simulink model "test_qdr_vacc4"  (Simulink 7.2)
settings: Solver=ode45  StartTime=0.0  StopTime=400000  RelTol=1e-3
libraries: xbsIndex_r4 x317, xps_library x15, casper_library_misc x4, casper_library_scopes x1
(part 2 of 3)

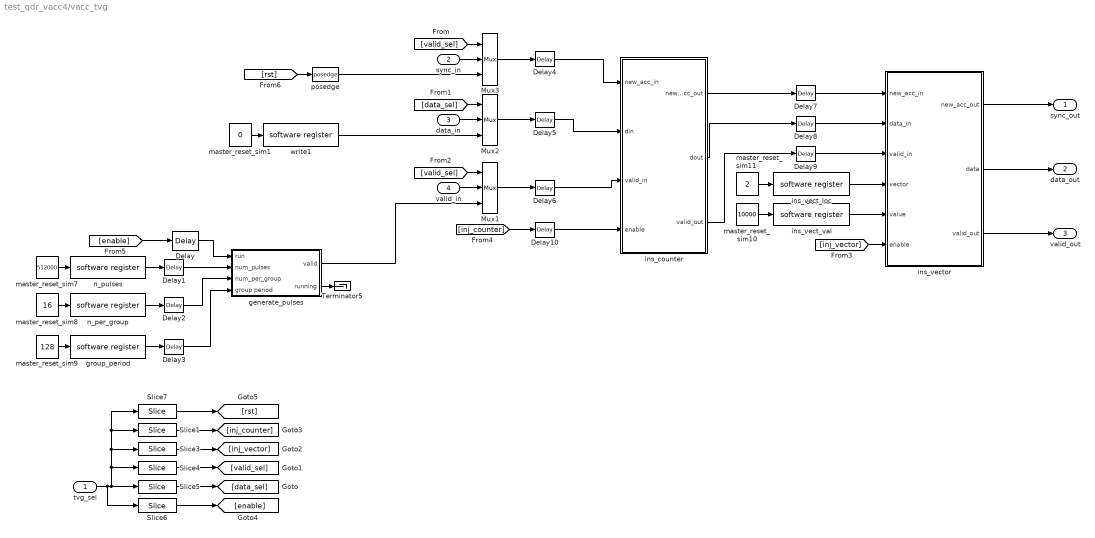
== system test_qdr_vacc4/vacc_tvg ==
  tvg_sel : Inport  OutDataType=sfix(16)  OutScaling=2^0
  sync_in : Inport  Port=2  OutDataType=sfix(16)  OutScaling=2^0
  data_in : Inport  Port=3  OutDataType=sfix(16)  OutScaling=2^0
  valid_in : Inport  Port=4  OutDataType=sfix(16)  OutScaling=2^0
  Delay : xbsIndex_r4/Delay  en=off  latency=1  dbl_ovrd=off  reg_retiming=on  block_type=delay
      settings: xl_area=[0, 0, 0, 0, 0, 0, 0]
  Delay{1..10} (10 alike) : xbsIndex_r4/Delay  en=off  latency=2  dbl_ovrd=off  reg_retiming=on  block_type=delay
  Mux1 : xbsIndex_r4/Mux  inputs=2  en=off  latency=0  precision=Full  arith_type="Signed  (2's comp)"  n_bits=8  bin_pt=2  quantization=Truncate  overflow=Wrap  dbl_ovrd=off  block_type=mux
      settings: xl_area=[0, 0, 0, 0, 0, 0, 0]
  Mux2 : xbsIndex_r4/Mux  inputs=2  en=off  latency=0  precision=Full  arith_type="Signed  (2's comp)"  n_bits=8  bin_pt=2  quantization=Truncate  overflow=Wrap  dbl_ovrd=off  block_type=mux
      settings: xl_area=[0, 0, 0, 0, 0, 0, 0]
  Mux3 : xbsIndex_r4/Mux  inputs=2  en=off  latency=0  precision=Full  arith_type="Signed  (2's comp)"  n_bits=8  bin_pt=2  quantization=Truncate  overflow=Wrap  dbl_ovrd=off  block_type=mux
      settings: xl_area=[0, 0, 0, 0, 0, 0, 0]
  Slice1 : xbsIndex_r4/Slice  nbits=1  boolean_output=on  mode=Lower Bit Location + Width  bit1=0  base1=MSB of Input  bit0=4  base0=LSB of Input  dbl_ovrd=off  block_type=slice
      settings: infoedit="Extracts a given range of bits from each input sample and presents it at the output.  The output type is ordinarily unsigned with binary point at zero, but can be Boolean when the slice is one bit wide.<P><P>Hardware notes: In hardware this block costs nothing."  block_version=10.1.3
  Slice3 : xbsIndex_r4/Slice  nbits=1  boolean_output=on  mode=Lower Bit Location + Width  bit1=0  base1=MSB of Input  bit0=3  base0=LSB of Input  dbl_ovrd=off  block_type=slice
      settings: infoedit="Extracts a given range of bits from each input sample and presents it at the output.  The output type is ordinarily unsigned with binary point at zero, but can be Boolean when the slice is one bit wide.<P><P>Hardware notes: In hardware this block costs nothing."  block_version=10.1.3
  Slice4 : xbsIndex_r4/Slice  nbits=1  boolean_output=on  mode=Lower Bit Location + Width  bit1=0  base1=MSB of Input  bit0=2  base0=LSB of Input  dbl_ovrd=off  block_type=slice
      settings: infoedit="Extracts a given range of bits from each input sample and presents it at the output.  The output type is ordinarily unsigned with binary point at zero, but can be Boolean when the slice is one bit wide.<P><P>Hardware notes: In hardware this block costs nothing."  block_version=10.1.3
  Slice5 : xbsIndex_r4/Slice  nbits=1  boolean_output=on  mode=Lower Bit Location + Width  bit1=0  base1=MSB of Input  bit0=1  base0=LSB of Input  dbl_ovrd=off  block_type=slice
      settings: infoedit="Extracts a given range of bits from each input sample and presents it at the output.  The output type is ordinarily unsigned with binary point at zero, but can be Boolean when the slice is one bit wide.<P><P>Hardware notes: In hardware this block costs nothing."  block_version=10.1.3
  Slice6 : xbsIndex_r4/Slice  nbits=1  boolean_output=on  mode=Lower Bit Location + Width  bit1=0  base1=MSB of Input  bit0=0  base0=LSB of Input  dbl_ovrd=off  block_type=slice
      settings: infoedit="Extracts a given range of bits from each input sample and presents it at the output.  The output type is ordinarily unsigned with binary point at zero, but can be Boolean when the slice is one bit wide.<P><P>Hardware notes: In hardware this block costs nothing."  block_version=10.1.3
  Slice7 : xbsIndex_r4/Slice  nbits=1  boolean_output=on  mode=Lower Bit Location + Width  bit1=0  base1=MSB of Input  bit0=5  base0=LSB of Input  dbl_ovrd=off  block_type=slice
      settings: infoedit="Extracts a given range of bits from each input sample and presents it at the output.  The output type is ordinarily unsigned with binary point at zero, but can be Boolean when the slice is one bit wide.<P><P>Hardware notes: In hardware this block costs nothing."  block_version=10.1.3
  Terminator5 : Terminator
  generate_pulses : Subsystem
  group_period : xps_library/software register  Tag=xps:sw_reg  SystemSampleTime=-1  io_dir=From Processor  arith_type=Unsigned  bitwidth=32  bin_pt=0  sample_period=1  gw_name=test_qdr_vacc4_vacc_tvg_group_period_user_data_out
      link override qdr_vacc_dram_tvg1_group_period_user_data_out: arith_type=Unsigned  n_bits=32  bin_pt=0  period=1
      link override qdr_vacc_qdr_tvg_group_period_user_data_out: arith_type=Unsigned  n_bits=32  bin_pt=0  period=1
      link override test_d_v_p_10_1_new_packet_format_qdr_tvg_group_period_user_data_out: arith_type=Unsigned  n_bits=32  bin_pt=0  period=1
      link override test_qdr_vacc2_vacc_tvg_group_period_user_data_out: arith_type=Unsigned  n_bits=32  bin_pt=0  period=1
      link override test_qdr_vacc3_vacc_tvg_group_period_user_data_out: arith_type=Unsigned  n_bits=32  bin_pt=0  period=1
      link override test_qdr_vacc_qdr_tvg_group_period_user_data_out: arith_type=Unsigned  n_bits=32  bin_pt=0  period=1
      link override test_qdr_vacc_vacc_tvg_group_period_user_data_out: arith_type=Unsigned  n_bits=32  bin_pt=0  period=1
      link override test_vacc_10_1_new_pkt_form_qdr_tvg_group_period_user_data_out: arith_type=Unsigned  n_bits=32  bin_pt=0  period=1
      link override test_vacc_pkt_10_1_vacc_tvg0_group_period_user_data_out: arith_type=Unsigned  n_bits=32  bin_pt=0  period=1
      link override test_vacc_pkt_10_1_vacc_tvg_group_period_user_data_out: arith_type=Unsigned  n_bits=32  bin_pt=0  period=1
      link override xflow_sim_8a_vacc_tvg0_group_period_user_data_out: arith_type=Unsigned  n_bits=32  bin_pt=0  period=1
      link override xflow_sim_vacc_tvg0_group_period_user_data_out: arith_type=Unsigned  n_bits=32  bin_pt=0  period=1
  ins_counter : Subsystem  mask{vec_len=len}
      mask prompts: vec_len "Vector Length?"
      mask init:
      | fmtstr = sprintf('Vector Length: %d', vec_len);
      | set_param(gcb, 'AttributesFormatString', fmtstr);
      settings: AttributesFormatString=Vector Length: 1000
  ins_vect_loc : xps_library/software register  Tag=xps:sw_reg  SystemSampleTime=-1  io_dir=From Processor  arith_type=Unsigned  bitwidth=32  bin_pt=0  sample_period=1  gw_name=test_qdr_vacc4_vacc_tvg_ins_vect_loc_user_data_out
      link override qdr_vacc_dram_tvg1_inject_vector_location_user_data_out: arith_type=Unsigned  n_bits=32  bin_pt=0  period=1
      link override qdr_vacc_qdr_tvg_inject_vector_location_user_data_out: arith_type=Unsigned  n_bits=32  bin_pt=0  period=1
      link override test_d_v_p_10_1_new_packet_format_qdr_tvg_inject_vector_location_user_data_out: arith_type=Unsigned  n_bits=32  bin_pt=0  period=1
      link override test_qdr_vacc2_vacc_tvg_ins_vect_loc_user_data_out: arith_type=Unsigned  n_bits=32  bin_pt=0  period=1
      link override test_qdr_vacc3_vacc_tvg_ins_vect_loc_user_data_out: arith_type=Unsigned  n_bits=32  bin_pt=0  period=1
      link override test_qdr_vacc_qdr_tvg_inject_vector_location_user_data_out: arith_type=Unsigned  n_bits=32  bin_pt=0  period=1
      link override test_qdr_vacc_vacc_tvg_ins_vect_loc_user_data_out: arith_type=Unsigned  n_bits=32  bin_pt=0  period=1
      link override test_vacc_10_1_new_pkt_form_qdr_tvg_inject_vector_location_user_data_out: arith_type=Unsigned  n_bits=32  bin_pt=0  period=1
      link override test_vacc_pkt_10_1_vacc_tvg0_ins_vect_loc_user_data_out: arith_type=Unsigned  n_bits=32  bin_pt=0  period=1
      link override test_vacc_pkt_10_1_vacc_tvg_inject_vector_location_user_data_out: arith_type=Unsigned  n_bits=32  bin_pt=0  period=1
      link override test_vacc_pkt_10_1_vacc_tvg_ins_vect_loc_user_data_out: arith_type=Unsigned  n_bits=32  bin_pt=0  period=1
      link override xflow_sim_8a_vacc_tvg0_ins_vect_loc_user_data_out: arith_type=Unsigned  n_bits=32  bin_pt=0  period=1
      link override xflow_sim_vacc_tvg0_ins_vect_loc_user_data_out: arith_type=Unsigned  n_bits=32  bin_pt=0  period=1
  ins_vect_val : xps_library/software register  Tag=xps:sw_reg  SystemSampleTime=-1  io_dir=From Processor  arith_type=Unsigned  bitwidth=32  bin_pt=0  sample_period=1  gw_name=test_qdr_vacc4_vacc_tvg_ins_vect_val_user_data_out
      link override qdr_vacc_dram_tvg1_inject_vector_value_user_data_out: arith_type=Unsigned  n_bits=32  bin_pt=0  period=1
      link override qdr_vacc_qdr_tvg_inject_vector_value_user_data_out: arith_type=Unsigned  n_bits=32  bin_pt=0  period=1
      link override test_d_v_p_10_1_new_packet_format_qdr_tvg_inject_vector_value_user_data_out: arith_type="Signed  (2's comp)"  n_bits=32  bin_pt=0  period=1
      link override test_qdr_vacc2_vacc_tvg_ins_vect_val_user_data_out: arith_type=Unsigned  n_bits=32  bin_pt=0  period=1
      link override test_qdr_vacc3_vacc_tvg_ins_vect_val_user_data_out: arith_type=Unsigned  n_bits=32  bin_pt=0  period=1
      link override test_qdr_vacc_qdr_tvg_inject_vector_value_user_data_out: arith_type="Signed  (2's comp)"  n_bits=32  bin_pt=0  period=1
      link override test_qdr_vacc_vacc_tvg_ins_vect_val_user_data_out: arith_type=Unsigned  n_bits=32  bin_pt=0  period=1
      link override test_vacc_10_1_new_pkt_form_qdr_tvg_inject_vector_value_user_data_out: arith_type="Signed  (2's comp)"  n_bits=32  bin_pt=0  period=1
      link override test_vacc_pkt_10_1_vacc_tvg0_ins_vect_val_user_data_out: arith_type=Unsigned  n_bits=32  bin_pt=0  period=1
      link override test_vacc_pkt_10_1_vacc_tvg_inject_vector_value_user_data_out: arith_type="Signed  (2's comp)"  n_bits=32  bin_pt=0  period=1
      link override test_vacc_pkt_10_1_vacc_tvg_ins_vect_val_user_data_out: arith_type="Signed  (2's comp)"  n_bits=32  bin_pt=0  period=1
      link override xflow_sim_8a_vacc_tvg0_ins_vect_val_user_data_out: arith_type=Unsigned  n_bits=32  bin_pt=0  period=1
      link override xflow_sim_vacc_tvg0_ins_vect_val_user_data_out: arith_type=Unsigned  n_bits=32  bin_pt=0  period=1
  ins_vector : Subsystem  mask{num_vectors=len}
      mask prompts: num_vectors "number of vectors"
      mask init:
      | fmtstr = sprintf('Vector Length: %d', num_vectors);
      | set_param(gcb, 'AttributesFormatString', fmtstr);
      settings: AttributesFormatString=Vector Length: 1000
  master_reset_sim1 : Constant  Value=0  OutDataType=sfix(16)  OutScaling=2^0
  master_reset_sim10 : Constant  Value=10000  OutDataType=sfix(16)  OutScaling=2^0
  master_reset_sim11 : Constant  Value=2  OutDataType=sfix(16)  OutScaling=2^0
  master_reset_sim7 : Constant  Value=512000  OutDataType=sfix(16)  OutScaling=2^0
  master_reset_sim8 : Constant  Value=16  OutDataType=sfix(16)  OutScaling=2^0
  master_reset_sim9 : Constant  Value=128  OutDataType=sfix(16)  OutScaling=2^0
  n_per_group : xps_library/software register  Tag=xps:sw_reg  SystemSampleTime=-1  io_dir=From Processor  arith_type=Unsigned  bitwidth=32  bin_pt=0  sample_period=1  gw_name=test_qdr_vacc4_vacc_tvg_n_per_group_user_data_out
      link override qdr_vacc_dram_tvg1_num_per_group_user_data_out: arith_type=Unsigned  n_bits=32  bin_pt=0  period=1
      link override qdr_vacc_qdr_tvg_num_per_group_user_data_out: arith_type=Unsigned  n_bits=32  bin_pt=0  period=1
      link override test_d_v_p_10_1_new_packet_format_qdr_tvg_num_per_group_user_data_out: arith_type=Unsigned  n_bits=32  bin_pt=0  period=1
      link override test_qdr_vacc2_vacc_tvg_n_per_group_user_data_out: arith_type=Unsigned  n_bits=32  bin_pt=0  period=1
      link override test_qdr_vacc3_vacc_tvg_n_per_group_user_data_out: arith_type=Unsigned  n_bits=32  bin_pt=0  period=1
      link override test_qdr_vacc_qdr_tvg_num_per_group_user_data_out: arith_type=Unsigned  n_bits=32  bin_pt=0  period=1
      link override test_qdr_vacc_vacc_tvg_n_per_group_user_data_out: arith_type=Unsigned  n_bits=32  bin_pt=0  period=1
      link override test_vacc_10_1_new_pkt_form_qdr_tvg_num_per_group_user_data_out: arith_type=Unsigned  n_bits=32  bin_pt=0  period=1
      link override test_vacc_pkt_10_1_vacc_tvg0_num_per_group_user_data_out: arith_type=Unsigned  n_bits=32  bin_pt=0  period=1
      link override test_vacc_pkt_10_1_vacc_tvg_num_per_group_user_data_out: arith_type=Unsigned  n_bits=32  bin_pt=0  period=1
      link override xflow_sim_8a_vacc_tvg0_num_per_group_user_data_out: arith_type=Unsigned  n_bits=32  bin_pt=0  period=1
      link override xflow_sim_vacc_tvg0_num_per_group_user_data_out: arith_type=Unsigned  n_bits=32  bin_pt=0  period=1
  n_pulses : xps_library/software register  Tag=xps:sw_reg  SystemSampleTime=-1  io_dir=From Processor  arith_type=Unsigned  bitwidth=32  bin_pt=0  sample_period=1  gw_name=test_qdr_vacc4_vacc_tvg_n_pulses_user_data_out
      link override qdr_vacc_dram_tvg1_num_pulses_user_data_out: arith_type=Unsigned  n_bits=32  bin_pt=0  period=1
      link override qdr_vacc_qdr_tvg_num_pulses_user_data_out: arith_type=Unsigned  n_bits=32  bin_pt=0  period=1
      link override test_d_v_p_10_1_new_packet_format_qdr_tvg_num_pulses_user_data_out: arith_type=Unsigned  n_bits=32  bin_pt=0  period=1
      link override test_qdr_vacc2_vacc_tvg_n_pulses_user_data_out: arith_type=Unsigned  n_bits=32  bin_pt=0  period=1
      link override test_qdr_vacc3_vacc_tvg_n_pulses_user_data_out: arith_type=Unsigned  n_bits=32  bin_pt=0  period=1
      link override test_qdr_vacc_qdr_tvg_num_pulses_user_data_out: arith_type=Unsigned  n_bits=32  bin_pt=0  period=1
      link override test_qdr_vacc_vacc_tvg_n_pulses_user_data_out: arith_type=Unsigned  n_bits=32  bin_pt=0  period=1
      link override test_vacc_10_1_new_pkt_form_qdr_tvg_num_pulses_user_data_out: arith_type=Unsigned  n_bits=32  bin_pt=0  period=1
      link override test_vacc_pkt_10_1_vacc_tvg0_num_pulses_user_data_out: arith_type=Unsigned  n_bits=32  bin_pt=0  period=1
      link override test_vacc_pkt_10_1_vacc_tvg_num_pulses_user_data_out: arith_type=Unsigned  n_bits=32  bin_pt=0  period=1
      link override xflow_sim_8a_vacc_tvg0_num_pulses_user_data_out: arith_type=Unsigned  n_bits=32  bin_pt=0  period=1
      link override xflow_sim_vacc_tvg0_num_pulses_user_data_out: arith_type=Unsigned  n_bits=32  bin_pt=0  period=1
  posedge : casper_library_misc/posedge  Tag=Rising Edge Detector  SystemSampleTime=-1
  write1 : xps_library/software register  Tag=xps:sw_reg  SystemSampleTime=-1  io_dir=From Processor  arith_type=Unsigned  bitwidth=32  bin_pt=0  sample_period=1  gw_name=test_qdr_vacc4_vacc_tvg_write1_user_data_out
      link override qdr_vacc_dram_tvg1_write1_user_data_out: arith_type=Unsigned  n_bits=32  bin_pt=0  period=1
      link override qdr_vacc_qdr_tvg_write1_user_data_out: arith_type=Unsigned  n_bits=32  bin_pt=0  period=1
      link override test_d_v_p_10_1_new_packet_format_qdr_tvg_write1_user_data_out: arith_type="Signed  (2's comp)"  n_bits=32  bin_pt=0  period=1
      link override test_qdr_vacc2_vacc_tvg_write1_user_data_out: arith_type=Unsigned  n_bits=32  bin_pt=0  period=1
      link override test_qdr_vacc3_vacc_tvg_write1_user_data_out: arith_type=Unsigned  n_bits=32  bin_pt=0  period=1
      link override test_qdr_vacc_qdr_tvg_write1_user_data_out: arith_type="Signed  (2's comp)"  n_bits=32  bin_pt=0  period=1
      link override test_qdr_vacc_vacc_tvg_write1_user_data_out: arith_type=Unsigned  n_bits=32  bin_pt=0  period=1
      link override test_vacc_10_1_new_pkt_form_qdr_tvg_write1_user_data_out: arith_type="Signed  (2's comp)"  n_bits=32  bin_pt=0  period=1
      link override test_vacc_pkt_10_1_vacc_tvg0_write1_user_data_out: arith_type=Unsigned  n_bits=32  bin_pt=0  period=1
      link override test_vacc_pkt_10_1_vacc_tvg_write1_user_data_out: arith_type="Signed  (2's comp)"  n_bits=32  bin_pt=0  period=1
      link override xflow_sim_8a_vacc_tvg0_write1_user_data_out: arith_type=Unsigned  n_bits=32  bin_pt=0  period=1
      link override xflow_sim_vacc_tvg0_write1_user_data_out: arith_type=Unsigned  n_bits=32  bin_pt=0  period=1
  sync_out : Outport  OutDataType=sfix(16)  OutScaling=2^0
  data_out : Outport  Port=2  OutDataType=sfix(16)  OutScaling=2^0
  valid_out : Outport  Port=3  OutDataType=sfix(16)  OutScaling=2^0
  wires:
  generate_pulses/2(running) -> Terminator5/1
  Delay/1 -> generate_pulses/1(run)
  Slice7/1 -> [rst]
  Slice6/1 -> [enable]
  [inj_counter] -> Delay10/1
  ins_vect_val/1 -> ins_vector/5(value)
  master_reset_sim10/1 -> ins_vect_val/1
  ins_vect_loc/1 -> ins_vector/4(vector)
  master_reset_sim11/1 -> ins_vect_loc/1
  [inj_vector] -> ins_vector/6(enable)
  posedge/1 -> Mux3/3
  generate_pulses/1(valid) -> Mux1/3
  ins_counter/3(valid_out) -> Delay9/1
  ins_counter/2(dout) -> Delay8/1
  [enable] -> Delay/1
  Slice1/1 -> [inj_counter]
  Slice3/1 -> [inj_vector]
  [valid_sel] -> Mux1/1
  [data_sel] -> Mux2/1
  [valid_sel] -> Mux3/1
  Slice4/1 -> [valid_sel]
  tvg_sel/1 -> Slice6/1, Slice4/1, Slice7/1, Slice1/1, Slice3/1, Slice5/1
  Slice5/1 -> [data_sel]
  Mux3/1 -> Delay4/1
  sync_in/1 -> Mux3/2
  data_in/1 -> Mux2/2
  Mux2/1 -> Delay5/1
  ins_counter/1(new_acc_out) -> Delay7/1
  ins_vector/3(valid_out) -> valid_out/1
  ins_vector/2(data) -> data_out/1
  ins_vector/1(new_acc_out) -> sync_out/1
  valid_in/1 -> Mux1/2
  Mux1/1 -> Delay6/1
  master_reset_sim9/1 -> group_period/1
  group_period/1 -> Delay3/1
  master_reset_sim8/1 -> n_per_group/1
  n_per_group/1 -> Delay2/1
  master_reset_sim7/1 -> n_pulses/1
  n_pulses/1 -> Delay1/1
  [rst] -> posedge/1
  master_reset_sim1/1 -> write1/1
  write1/1 -> Mux2/3
  Delay1/1 -> generate_pulses/2(num_pulses)
  Delay2/1 -> generate_pulses/3(num_per_group)
  Delay3/1 -> generate_pulses/4(group period)
  Delay4/1 -> ins_counter/1(new_acc_in)
  Delay5/1 -> ins_counter/2(din)
  Delay6/1 -> ins_counter/3(valid_in)
  Delay7/1 -> ins_vector/1(new_acc_in)
  Delay8/1 -> ins_vector/2(data_in)
  Delay9/1 -> ins_vector/3(valid_in)
  Delay10/1 -> ins_counter/4(enable)

== system test_qdr_vacc4/Subsystem/data_sel1 ==
  In1 : Inport  OutDataType=sfix(16)  OutScaling=2^0
  Product : Product  OutDataType=sfix(16)  OutScaling=2^0  RndMeth=Zero
  err_clear_sim1 : Constant  Value=2^bit_pos  OutDataType=sfix(16)  OutScaling=2^0
  Out1 : Outport  OutDataType=sfix(16)  OutScaling=2^0
  wires:
  err_clear_sim1/1 -> Product/2
  In1/1 -> Product/1
  Product/1 -> Out1/1

== system test_qdr_vacc4/Subsystem/inj_counter1 ==
  In1 : Inport  OutDataType=sfix(16)  OutScaling=2^0
  Product : Product  OutDataType=sfix(16)  OutScaling=2^0  RndMeth=Zero
  err_clear_sim1 : Constant  Value=2^bit_pos  OutDataType=sfix(16)  OutScaling=2^0
  Out1 : Outport  OutDataType=sfix(16)  OutScaling=2^0
  wires:
  err_clear_sim1/1 -> Product/2
  In1/1 -> Product/1
  Product/1 -> Out1/1

== system test_qdr_vacc4/Subsystem/inj_vector1 ==
  In1 : Inport  OutDataType=sfix(16)  OutScaling=2^0
  Product : Product  OutDataType=sfix(16)  OutScaling=2^0  RndMeth=Zero
  err_clear_sim1 : Constant  Value=2^bit_pos  OutDataType=sfix(16)  OutScaling=2^0
  Out1 : Outport  OutDataType=sfix(16)  OutScaling=2^0
  wires:
  err_clear_sim1/1 -> Product/2
  In1/1 -> Product/1
  Product/1 -> Out1/1

== system test_qdr_vacc4/Subsystem/new_acc2 ==
  In1 : Inport  OutDataType=sfix(16)  OutScaling=2^0
  Product : Product  OutDataType=sfix(16)  OutScaling=2^0  RndMeth=Zero
  err_clear_sim1 : Constant  Value=2^bit_pos  OutDataType=sfix(16)  OutScaling=2^0
  Out1 : Outport  OutDataType=sfix(16)  OutScaling=2^0
  wires:
  err_clear_sim1/1 -> Product/2
  In1/1 -> Product/1
  Product/1 -> Out1/1

== system test_qdr_vacc4/Subsystem/run1 ==
  In1 : Inport  OutDataType=sfix(16)  OutScaling=2^0
  Product : Product  OutDataType=sfix(16)  OutScaling=2^0  RndMeth=Zero
  err_clear_sim1 : Constant  Value=2^bit_pos  OutDataType=sfix(16)  OutScaling=2^0
  Out1 : Outport  OutDataType=sfix(16)  OutScaling=2^0
  wires:
  err_clear_sim1/1 -> Product/2
  In1/1 -> Product/1
  Product/1 -> Out1/1

== system test_qdr_vacc4/Subsystem/valid_sel1 ==
  In1 : Inport  OutDataType=sfix(16)  OutScaling=2^0
  Product : Product  OutDataType=sfix(16)  OutScaling=2^0  RndMeth=Zero
  err_clear_sim1 : Constant  Value=2^bit_pos  OutDataType=sfix(16)  OutScaling=2^0
  Out1 : Outport  OutDataType=sfix(16)  OutScaling=2^0
  wires:
  err_clear_sim1/1 -> Product/2
  In1/1 -> Product/1
  Product/1 -> Out1/1

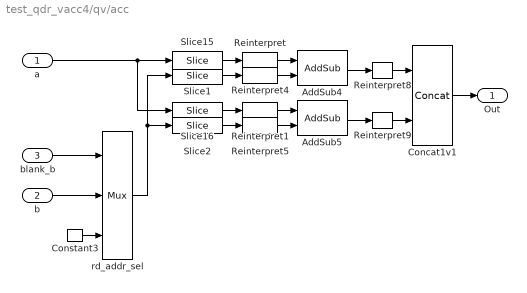
== system test_qdr_vacc4/qv/acc ==
  a : Inport
  b : Inport  Port=2
  blank_b : Inport  Port=3
  AddSub4 : xbsIndex_r4/AddSub  mode=Addition  use_carryin=off  use_carryout=off  en=off  latency=2  precision=User Defined  arith_type="Signed  (2's comp)"  n_bits=4  bin_pt=0  quantization="Round  (unbiased: +/- Inf)"  overflow=Wrap  dbl_ovrd=off  use_behavioral_HDL=on  hw_selection=Fabric  pipelined=on  use_rpm=on  block_type=addsub
      settings: xl_area=[0, 0, 0, 0, 0, 0, 0]  block_version=9.2.01
  AddSub5 : xbsIndex_r4/AddSub  mode=Addition  use_carryin=off  use_carryout=off  en=off  latency=2  precision=User Defined  arith_type="Signed  (2's comp)"  n_bits=32  bin_pt=0  quantization="Round  (unbiased: +/- Inf)"  overflow=Wrap  dbl_ovrd=off  use_behavioral_HDL=on  hw_selection=Fabric  pipelined=on  use_rpm=on  block_type=addsub
      settings: xl_area=[0, 0, 0, 0, 0, 0, 0]  block_version=9.2.01
  Concat1v1 : xbsIndex_r4/Concat  num_inputs=2  dbl_ovrd=off  block_type=concat
      settings: block_version=9.2.01
  Constant3 : xbsIndex_r4/Constant  arith_type=Unsigned  const=0  n_bits=36  bin_pt=0  explicit_period=on  period=1  equ=P=C  opselect=C  inp2=PCIN>>17  opr=+  inp1=P  carry=CIN  dbl_ovrd=off  block_type=constant
      settings: block_version=9.2.01
  Reinterpret{,1,4..5} (4 alike) : xbsIndex_r4/Reinterpret  force_arith_type=on  arith_type="Signed  (2's comp)"  force_bin_pt=on  bin_pt=0  block_type=reinterpret
      settings: infoedit="Changes signal type without altering the binary representation.   You can changed the signal between signed and unsigned, and relocate the binary point.<P><P>Hardware notes: In hardware this block costs nothing.<P><P>Example:  Suppose the input is 6 bits wide, signed, with 2 fractional bits, and the output is forced to unsigned with 0 fractional bits.  Then an input of -2.0 (1110.00 in binary 2's complement) becomes an output of 56 (111000 in binary)."  block_version=9.2.01
  Reinterpret8 : xbsIndex_r4/Reinterpret  force_arith_type=on  arith_type=Unsigned  force_bin_pt=on  bin_pt=0  block_type=reinterpret
      settings: infoedit="Changes signal type without altering the binary representation.   You can changed the signal between signed and unsigned, and relocate the binary point.<P><P>Hardware notes: In hardware this block costs nothing.<P><P>Example:  Suppose the input is 6 bits wide, signed, with 2 fractional bits, and the output is forced to unsigned with 0 fractional bits.  Then an input of -2.0 (1110.00 in binary 2's complement) becomes an output of 56 (111000 in binary)."  block_version=9.2.01
  Reinterpret9 : xbsIndex_r4/Reinterpret  force_arith_type=on  arith_type=Unsigned  force_bin_pt=on  bin_pt=0  block_type=reinterpret
      settings: infoedit="Changes signal type without altering the binary representation.   You can changed the signal between signed and unsigned, and relocate the binary point.<P><P>Hardware notes: In hardware this block costs nothing.<P><P>Example:  Suppose the input is 6 bits wide, signed, with 2 fractional bits, and the output is forced to unsigned with 0 fractional bits.  Then an input of -2.0 (1110.00 in binary 2's complement) becomes an output of 56 (111000 in binary)."  block_version=9.2.01
  Slice1 : xbsIndex_r4/Slice  nbits=4  boolean_output=off  mode=Lower Bit Location + Width  bit1=96  base1=MSB of Input  bit0=32  base0=LSB of Input  dbl_ovrd=off  block_type=slice
      settings: infoedit="Extracts a given range of bits from each input sample and presents it at the output.  The output type is ordinarily unsigned with binary point at zero, but can be Boolean when the slice is one bit wide.<P><P>Hardware notes: In hardware this block costs nothing."  block_version=9.2.01
  Slice15 : xbsIndex_r4/Slice  nbits=4  boolean_output=off  mode=Lower Bit Location + Width  bit1=96  base1=MSB of Input  bit0=32  base0=LSB of Input  dbl_ovrd=off  block_type=slice
      settings: infoedit="Extracts a given range of bits from each input sample and presents it at the output.  The output type is ordinarily unsigned with binary point at zero, but can be Boolean when the slice is one bit wide.<P><P>Hardware notes: In hardware this block costs nothing."  block_version=9.2.01
  Slice16 : xbsIndex_r4/Slice  nbits=32  boolean_output=off  mode=Lower Bit Location + Width  bit1=-32  base1=MSB of Input  bit0=0  base0=LSB of Input  dbl_ovrd=off  block_type=slice
      settings: infoedit="Extracts a given range of bits from each input sample and presents it at the output.  The output type is ordinarily unsigned with binary point at zero, but can be Boolean when the slice is one bit wide.<P><P>Hardware notes: In hardware this block costs nothing."  block_version=9.2.01
  Slice2 : xbsIndex_r4/Slice  nbits=32  boolean_output=off  mode=Lower Bit Location + Width  bit1=-32  base1=MSB of Input  bit0=0  base0=LSB of Input  dbl_ovrd=off  block_type=slice
      settings: infoedit="Extracts a given range of bits from each input sample and presents it at the output.  The output type is ordinarily unsigned with binary point at zero, but can be Boolean when the slice is one bit wide.<P><P>Hardware notes: In hardware this block costs nothing."  block_version=9.2.01
  rd_addr_sel : xbsIndex_r4/Mux  inputs=2  en=off  latency=0  precision=Full  arith_type=Unsigned  n_bits=16  bin_pt=14  quantization=Truncate  overflow=Wrap  dbl_ovrd=off  block_type=mux
  Out : Outport
  wires:
  Reinterpret8/1 -> Concat1v1/1
  Reinterpret/1 -> AddSub4/1
  Slice15/1 -> Reinterpret/1
  Slice1/1 -> Reinterpret4/1
  Reinterpret4/1 -> AddSub4/2
  AddSub4/1 -> Reinterpret8/1
  a/1 -> Slice15/1, Slice16/1
  Concat1v1/1 -> Out/1
  Reinterpret9/1 -> Concat1v1/2
  Reinterpret1/1 -> AddSub5/1
  Slice16/1 -> Reinterpret1/1
  Slice2/1 -> Reinterpret5/1
  Reinterpret5/1 -> AddSub5/2
  AddSub5/1 -> Reinterpret9/1
  b/1 -> rd_addr_sel/2
  rd_addr_sel/1 -> Slice2/1, Slice1/1
  blank_b/1 -> rd_addr_sel/1
  Constant3/1 -> rd_addr_sel/3

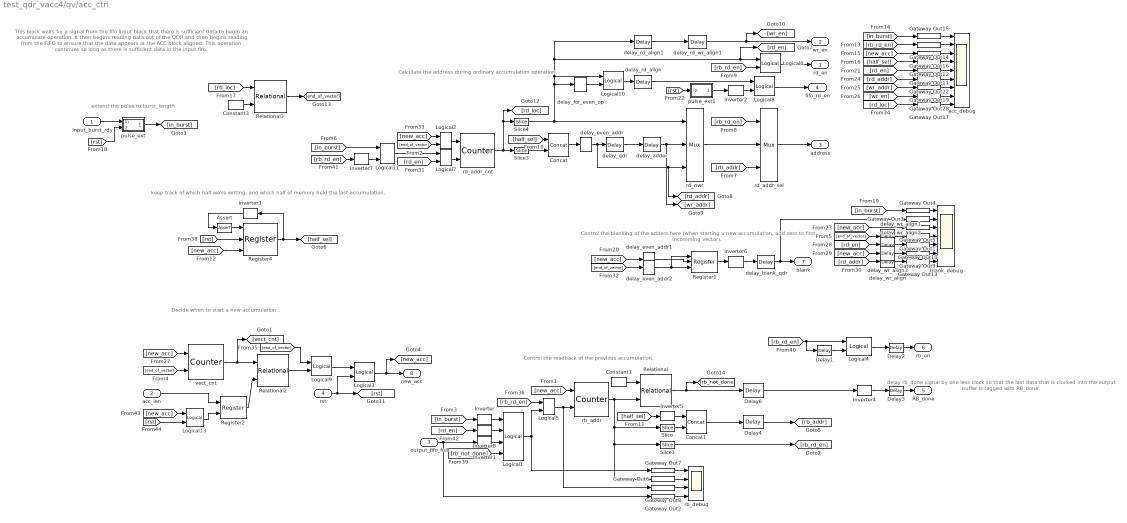
== system test_qdr_vacc4/qv/acc_ctrl ==
  note: Decide when to start a new accumulation.
  note: Calculate the address during ordinary
      | accumulation operation.
  note: Control the blanking of the
      | adders here (when starting a
      | new accumulation, add zero
      | to first incomming vector).
  note: Control the readback of the
      | previous accumulation.
  note: delay rb_done signal by
      | one less clock so that the last
      | data that is clocked into
      | the output buffer is tagged with RB_done
  note: keep track of which half we're writing,
      | and which half of memory
      | held the last accumulation.
  note: This block waits for a signal from the
      | fifo input block that there is sufficient data
      | to begin an accumulate operation.
      |
      | It then begins reading data out of the QDR and
      | then begins reading from the FIFO to ensure
      | that the data appears at the ACC block aligned.
      |
      | This operation continues so long as there is
      | sufficient data in the input fifo.
  note: extend the pulse to
      | burst_length
  input_burst_rdy : Inport  OutDataType=sfix(16)  OutScaling=2^0
  acc_len : Inport  Port=2  OutDataType=sfix(16)  OutScaling=2^0
  output_fifo_full : Inport  Port=3  OutDataType=sfix(16)  OutScaling=2^0
  rst : Inport  Port=4  OutDataType=sfix(16)  OutScaling=2^0
  Assert : xbsIndex_r4/Assert  assert_type=on  type_source=Explicitly  arith_type=Unsigned  n_bits=1  bin_pt=0  assert_rate=on  rate_source=Explicitly  period=1  output_port=on  block_type=assert
      settings: infoedit=Asserts a user-defined sample rate and/or type on a signal.<P><P>Hardware notes: In hardware this block costs nothing.  block_version=10.1.3
  Concat : xbsIndex_r4/Concat  num_inputs=2  dbl_ovrd=off  block_type=concat
      settings: block_version=10.1.3
  Concat1 : xbsIndex_r4/Concat  num_inputs=2  dbl_ovrd=off  block_type=concat
      settings: block_version=10.1.3
  Constant1 : xbsIndex_r4/Constant  arith_type=Unsigned  const=vector_len - 1  n_bits=vector_bits  bin_pt=0  explicit_period=on  period=1  equ=P=C  opselect=C  inp2=PCIN>>17  opr=+  inp1=P  carry=CIN  dbl_ovrd=off  block_type=constant
  Constant3 : xbsIndex_r4/Constant  arith_type=Unsigned  const=vector_len-1  n_bits=vector_bits  bin_pt=0  explicit_period=on  period=1  equ=P=C  opselect=C  inp2=PCIN>>17  opr=+  inp1=P  carry=CIN  dbl_ovrd=off  block_type=constant
  Delay1 : xbsIndex_r4/Delay  en=off  latency=1  dbl_ovrd=off  reg_retiming=on  block_type=delay
  Delay2 : xbsIndex_r4/Delay  en=off  latency=delay_qdr  dbl_ovrd=off  reg_retiming=on  block_type=delay
  Delay3 : xbsIndex_r4/Delay  en=off  latency=delay_qdr-1  dbl_ovrd=off  reg_retiming=on  block_type=delay
  Delay4 : xbsIndex_r4/Delay  en=off  latency=1  dbl_ovrd=off  reg_retiming=on  block_type=delay
  Delay6 : xbsIndex_r4/Delay  en=off  latency=1  dbl_ovrd=off  reg_retiming=on  block_type=delay
  Gateway Out{1..17,19,22,28} (20 alike) : xbsIndex_r4/Gateway Out  hdl_port=off  timing_constraint=None  locs_specified=off  LOCs={}  block_type=gatewayout
      settings: infoedit="Gateway out block.  Converts Xilinx fixed point inputs into ouputs of type Simulink integer, double, or fixed point.<P><P>Hardware notes:  In hardware these blocks become top level output ports or are discarded, depending on how they are configured."  xl_area=[0, 0, 0, 0, 0, 0, 0]  block_version=10.1.3
  Inverter{,1..2,4..8} (8 alike) : xbsIndex_r4/Inverter  en=off  latency=0  dbl_ovrd=off  block_type=inv
  Inverter3 : xbsIndex_r4/Inverter  Orientation=left  en=off  latency=0  dbl_ovrd=off  block_type=inv
  Logical1 : xbsIndex_r4/Logical  logical_function=AND  inputs=4  en=off  latency=0  precision=Full  arith_type=Unsigned  n_bits=16  bin_pt=0  align_bp=on  dbl_ovrd=off  block_type=logical
  Logical{2..7,10,13} (8 alike) : xbsIndex_r4/Logical  logical_function=OR  inputs=2  en=off  latency=0  precision=Full  arith_type=Unsigned  n_bits=16  bin_pt=0  align_bp=on  dbl_ovrd=off  block_type=logical
  Logical11 : xbsIndex_r4/Logical  logical_function=AND  inputs=2  en=off  latency=0  precision=Full  arith_type=Unsigned  n_bits=16  bin_pt=0  align_bp=on  dbl_ovrd=off  block_type=logical
  Logical8 : xbsIndex_r4/Logical  logical_function=AND  inputs=2  en=off  latency=0  precision=Full  arith_type=Unsigned  n_bits=16  bin_pt=0  align_bp=on  dbl_ovrd=off  block_type=logical
  Logical9 : xbsIndex_r4/Logical  logical_function=AND  inputs=2  en=off  latency=0  precision=Full  arith_type=Unsigned  n_bits=16  bin_pt=0  align_bp=on  dbl_ovrd=off  block_type=logical
  Register1 : xbsIndex_r4/Register  init=0  rst=on  en=on  dbl_ovrd=off  block_type=register
  Register2 : xbsIndex_r4/Register  init=0  rst=off  en=on  dbl_ovrd=off  block_type=register
  Register4 : xbsIndex_r4/Register  init=0  rst=on  en=on  dbl_ovrd=off  block_type=register
  Relational : xbsIndex_r4/Relational  mode=a>=b  en=off  latency=0  dbl_ovrd=off  block_type=relational
      settings: block_version=10.1.3
  Relational2 : xbsIndex_r4/Relational  mode=a>=b  en=off  latency=0  dbl_ovrd=off  block_type=relational
      settings: block_version=10.1.3
  Relational3 : xbsIndex_r4/Relational  mode=a>=b  en=off  latency=0  dbl_ovrd=off  block_type=relational
      settings: block_version=10.1.3
  Slice : xbsIndex_r4/Slice  nbits=vector_bits-1  boolean_output=off  mode=Lower Bit Location + Width  bit1=0  base1=MSB of Input  bit0=1  base0=LSB of Input  dbl_ovrd=off  block_type=slice
      settings: infoedit="Extracts a given range of bits from each input sample and presents it at the output.  The output type is ordinarily unsigned with binary point at zero, but can be Boolean when the slice is one bit wide.<P><P>Hardware notes: In hardware this block costs nothing."  block_version=10.1.3
  Slice1 : xbsIndex_r4/Slice  nbits=1  boolean_output=on  mode=Lower Bit Location + Width  bit1=-1  base1=MSB of Input  bit0=0  base0=LSB of Input  dbl_ovrd=off  block_type=slice
      settings: infoedit="Extracts a given range of bits from each input sample and presents it at the output.  The output type is ordinarily unsigned with binary point at zero, but can be Boolean when the slice is one bit wide.<P><P>Hardware notes: In hardware this block costs nothing."  block_version=10.1.3
  Slice3 : xbsIndex_r4/Slice  nbits=1  boolean_output=off  mode=Two Bit Locations  bit1=0  base1=MSB of Input  bit0=1  base0=LSB of Input  dbl_ovrd=off  block_type=slice
      settings: infoedit="Extracts a given range of bits from each input sample and presents it at the output.  The output type is ordinarily unsigned with binary point at zero, but can be Boolean when the slice is one bit wide.<P><P>Hardware notes: In hardware this block costs nothing."  block_version=10.1.3
  Slice4 : xbsIndex_r4/Slice  nbits=1  boolean_output=on  mode=Lower Bit Location + Width  bit1=-1  base1=MSB of Input  bit0=0  base0=LSB of Input  dbl_ovrd=off  block_type=slice
      settings: infoedit="Extracts a given range of bits from each input sample and presents it at the output.  The output type is ordinarily unsigned with binary point at zero, but can be Boolean when the slice is one bit wide.<P><P>Hardware notes: In hardware this block costs nothing."  block_version=10.1.3
  acc_debug : Scope  NumInputPorts=9
      settings: TimeRange=10000  YMin=0~-1~-1~0.95~0~500~500~0~-5  YMax=1~1~1~1.05~1~1100~1100~1~5  SaveName=ScopeData5
  blank_debug : Scope  NumInputPorts=7
      settings: TimeRange=10000  YMin=0~1~-1~-1~0~-1~50  YMax=1~1~1~1~1~1~250  SaveName=ScopeData6
  delay_adder : xbsIndex_r4/Delay  en=off  latency=delay_adder  dbl_ovrd=off  reg_retiming=off  block_type=delay
  delay_blank_qdr : xbsIndex_r4/Delay  en=off  latency=delay_qdr  dbl_ovrd=off  reg_retiming=on  block_type=delay
  delay_even_addr : xbsIndex_r4/Delay  en=off  latency=1  dbl_ovrd=off  reg_retiming=on  block_type=delay
  delay_even_addr1 : xbsIndex_r4/Delay  en=off  latency=1  dbl_ovrd=off  reg_retiming=on  block_type=delay
  delay_even_addr2 : xbsIndex_r4/Delay  en=off  latency=1  dbl_ovrd=off  reg_retiming=on  block_type=delay
  delay_for_even_op : xbsIndex_r4/Delay  en=off  latency=1  dbl_ovrd=off  reg_retiming=on  block_type=delay
  delay_qdr : xbsIndex_r4/Delay  en=off  latency=delay_qdr  dbl_ovrd=off  reg_retiming=off  block_type=delay
  delay_rd_align : xbsIndex_r4/Delay  en=off  latency=delay_qdr-delay_in_fifo  dbl_ovrd=off  reg_retiming=off  block_type=delay
  delay_rd_align1 : xbsIndex_r4/Delay  en=off  latency=delay_qdr  dbl_ovrd=off  reg_retiming=off  block_type=delay
  delay_rd_wr_align1 : xbsIndex_r4/Delay  en=off  latency=delay_adder  dbl_ovrd=off  reg_retiming=off  block_type=delay
  delay_wr_align{,1..3} (4 alike) : xbsIndex_r4/Delay  en=off  latency=delay_qdr  dbl_ovrd=off  reg_retiming=off  block_type=delay
  pulse_ext : Subsystem  AncestorBlock=casper_library/Misc/pulse_ext  mask(pulse_ext){pulse_len=burst_len}
      mask prompts: pulse_len "Length of Pulse"
      mask help:
      | Extends a boolean signal to be high for the specified number of clocks after
      | the last high input.
      mask init:
      | bits = ceil(log2(pulse_len+1));
      mask Help: eval('xlWeb([getenv(''MLIB_ROOT''), ''\doc\htmlblocks\sp_pulse_ext\sp_pulse_ext.html''])')
  pulse_ext1 : Subsystem  AncestorBlock=casper_library/Misc/pulse_ext  mask(pulse_ext){pulse_len=delay_qdr-delay_in_fifo}
      mask prompts: pulse_len "Length of Pulse"
      mask help:
      | Extends a boolean signal to be high for the specified number of clocks after
      | the last high input.
      mask init:
      | bits = ceil(log2(pulse_len+1));
      mask Help: eval('xlWeb([getenv(''MLIB_ROOT''), ''\doc\htmlblocks\sp_pulse_ext\sp_pulse_ext.html''])')
  rb_addr : xbsIndex_r4/Counter  cnt_type=Free Running  cnt_to=Inf  operation=Up  start_count=0  cnt_by_val=1  arith_type=Unsigned  n_bits=vector_bits  bin_pt=0  load_pin=off  rst=on  en=on  explicit_period=on  period=1  dbl_ovrd=off  use_behavioral_HDL=off  implementation=Fabric  use_rpm=off  block_type=counter
  rb_debug : Scope  NumInputPorts=4
      settings: TimeRange=10000  YMin=0~0~0~0  YMax=1~1000~1~1  SaveName=ScopeData5
  rd_addr_cnt : xbsIndex_r4/Counter  cnt_type=Free Running  cnt_to=vector_len-1  operation=Up  start_count=0  cnt_by_val=1  arith_type=Unsigned  n_bits=vector_bits  bin_pt=0  load_pin=off  rst=on  en=on  explicit_period=on  period=1  dbl_ovrd=off  use_behavioral_HDL=off  implementation=Fabric  use_rpm=off  block_type=counter
  rd_addr_sel : xbsIndex_r4/Mux  inputs=2  en=off  latency=0  precision=Full  arith_type=Unsigned  n_bits=16  bin_pt=14  quantization=Truncate  overflow=Wrap  dbl_ovrd=off  block_type=mux
  rd_nwr : xbsIndex_r4/Mux  inputs=2  en=off  latency=0  precision=Full  arith_type=Unsigned  n_bits=16  bin_pt=14  quantization=Truncate  overflow=Wrap  dbl_ovrd=off  block_type=mux
  vect_cnt : xbsIndex_r4/Counter  cnt_type=Free Running  cnt_to=Inf  operation=Up  start_count=1  cnt_by_val=1  arith_type=Unsigned  n_bits=32  bin_pt=0  load_pin=off  rst=on  en=on  explicit_period=on  period=1  dbl_ovrd=off  use_behavioral_HDL=off  implementation=Fabric  use_rpm=off  block_type=counter
  rd_en : Outport  OutDataType=sfix(16)  OutScaling=2^0
  wr_en : Outport  Port=2  OutDataType=sfix(16)  OutScaling=2^0
  address : Outport  Port=3  OutDataType=sfix(16)  OutScaling=2^0
  fifo_rd_en : Outport  Port=4  OutDataType=sfix(16)  OutScaling=2^0
  RB_done : Outport  Port=5  OutDataType=sfix(16)  OutScaling=2^0
  rb_en : Outport  Port=6  OutDataType=sfix(16)  OutScaling=2^0
  blank : Outport  Port=7  OutDataType=sfix(16)  OutScaling=2^0
  new_acc : Outport  Port=8  OutDataType=sfix(16)  OutScaling=2^0
  wires:
  Gateway Out1/1 -> blank_debug/4
  Logical5/1 -> rb_addr/2, Gateway Out8/1
  Delay1/1 -> Logical4/2
  Logical4/1 -> Delay2/1
  Delay6/1 -> Inverter4/1
  Logical1/1 -> Gateway Out7/1, Logical5/2
  delay_rd_wr_align1/1 -> [wr_en], wr_en/1
  delay_rd_align1/1 -> delay_rd_wr_align1/1
  Delay4/1 -> [rb_addr]
  Inverter4/1 -> Delay3/1
  rb_addr/1 -> Relational/2, Slice/1, Gateway Out6/1, Slice1/1
  Constant1/1 -> Relational/1
  Slice/1 -> Concat1/2
  Concat1/1 -> Delay4/1
  [rb_addr] -> rd_addr_sel/3
  Inverter5/1 -> Concat1/1
  [half_sel] -> Inverter5/1
  Concat/1 -> delay_even_addr/1
  [half_sel] -> Concat/1
  Delay3/1 -> RB_done/1
  Register2/1 -> Relational2/2
  [new_acc] -> vect_cnt/1
  Logical3/1 -> [new_acc], new_acc/1
  rst/1 -> [rst], Logical3/2
  Gateway Out28/1 -> acc_debug/8
  [wr_en] -> Gateway Out28/1
  delay_blank_qdr/1 -> Gateway Out3/1, blank/1
  Relational3/1 -> [end_of_vector]
  Constant3/1 -> Relational3/2
  [rd_loc] -> Relational3/1
  vect_cnt/1 -> Relational2/1, [vect_cnt]
  [wr_addr] -> Gateway Out19/1
  [rd_addr] -> Gateway Out22/1
  Gateway Out19/1 -> acc_debug/7
  Gateway Out22/1 -> acc_debug/6
  [rd_en] -> Gateway Out11/1
  [new_acc] -> Gateway Out5/1
  [in_burst] -> Gateway Out4/1
  Gateway Out5/1 -> blank_debug/3
  Gateway Out3/1 -> blank_debug/2
  Gateway Out4/1 -> blank_debug/1
  Register1/1 -> Inverter6/1
  [half_sel] -> Gateway Out12/1
  [new_acc] -> Gateway Out16/1
  [in_burst] -> Gateway Out15/1
  [rb_rd_en] -> Gateway Out14/1
  Gateway Out11/1 -> acc_debug/5
  Gateway Out12/1 -> acc_debug/4
  Gateway Out16/1 -> acc_debug/3
  Gateway Out14/1 -> acc_debug/2
  Gateway Out15/1 -> acc_debug/1
  Assert/1 -> Register4/1
  Inverter3/1 -> Assert/1
  Register4/1 -> [half_sel], Inverter3/1
  rd_addr_sel/1 -> address/1
  [rb_rd_en] -> Logical6/2
  rd_nwr/1 -> rd_addr_sel/2
  [rb_rd_en] -> rd_addr_sel/1
  [in_burst] -> Inverter/1
  Logical6/1 -> rd_en/1
  Delay2/1 -> rb_en/1
  output_fifo_full/1 -> Inverter1/1, Gateway Out2/1
  [new_acc] -> rb_addr/1
  Relational/1 -> Delay6/1, [rb_not_done]
  delay_adder/1 -> [wr_addr], rd_nwr/2
  delay_qdr/1 -> delay_adder/1
  rd_addr_cnt/1 -> Slice3/1, Slice4/1, [rd_loc]
  pulse_ext/1(out) -> [in_burst]
  input_burst_rdy/1 -> pulse_ext/1(in)
  Slice4/1 -> rd_nwr/1, delay_for_even_op/1, [rd_en], Logical6/1, delay_rd_align1/1, Logical10/1
  [rst] -> pulse_ext/2(rst)
  Gateway Out2/1 -> rb_debug/4
  Gateway Out8/1 -> rb_debug/3
  Gateway Out6/1 -> rb_debug/2
  Gateway Out7/1 -> rb_debug/1
  Gateway Out10/1 -> blank_debug/5
  Gateway Out9/1 -> blank_debug/6
  [rd_en] -> delay_wr_align2/1
  [new_acc] -> delay_wr_align3/1
  [rd_addr] -> delay_wr_align/1
  delay_wr_align/1 -> Gateway Out13/1
  Gateway Out13/1 -> blank_debug/7
  Slice3/1 -> Concat/2
  Logical7/1 -> rd_addr_cnt/2
  Logical11/1 -> Logical7/1
  [rd_en] -> Logical7/2
  [end_of_vector] -> vect_cnt/2
  [end_of_vector] -> delay_even_addr2/1
  [new_acc] -> delay_even_addr1/1
  [end_of_vector] -> delay_wr_align1/1
  Logical2/1 -> rd_addr_cnt/1
  [end_of_vector] -> Logical2/2
  [new_acc] -> Logical2/1
  Inverter6/1 -> delay_blank_qdr/1
  delay_wr_align1/1 -> Gateway Out1/1
  delay_wr_align3/1 -> Gateway Out9/1
  delay_wr_align2/1 -> Gateway Out10/1
  [rd_loc] -> Gateway Out17/1
  Gateway Out17/1 -> acc_debug/9
  Relational2/1 -> Logical9/2
  Logical9/1 -> Logical3/1
  [end_of_vector] -> Logical9/1
  Slice1/1 -> [rb_rd_en]
  delay_even_addr/1 -> [rd_addr], rd_nwr/3, delay_qdr/1
  delay_even_addr1/1 -> Register1/2
  delay_even_addr2/1 -> Register1/1, Register1/3
  [new_acc] -> Register4/3
  [rst] -> Register4/2
  delay_rd_align/1 -> Logical8/1
  Logical8/1 -> fifo_rd_en/1
  [rst] -> pulse_ext1/1(in)
  Inverter2/1 -> Logical8/2
  pulse_ext1/1(out) -> Inverter2/1
  Logical10/1 -> delay_rd_align/1
  delay_for_even_op/1 -> Logical10/2
  [rb_rd_en] -> Logical4/1, Delay1/1
  [rb_rd_en] -> Logical5/1
  [rb_rd_en] -> Inverter7/1
  [in_burst] -> Logical11/1
  Inverter/1 -> Logical1/1
  Inverter1/1 -> Logical1/3
  [rb_not_done] -> Logical1/4
  Inverter7/1 -> Logical11/2
  [rd_en] -> Inverter8/1
  Inverter8/1 -> Logical1/2
  [new_acc] -> Logical13/1
  [rst] -> Logical13/2
  acc_len/1 -> Register2/1
  Logical13/1 -> Register2/2

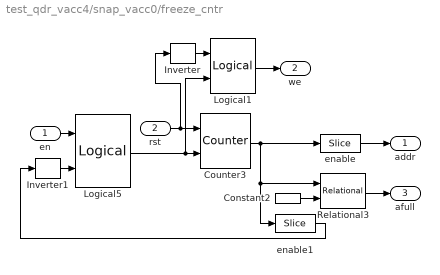
== system test_qdr_vacc4/snap_vacc0/freeze_cntr ==
  en : Inport  OutDataType=sfix(16)  OutScaling=2^0
  rst : Inport  Port=2  OutDataType=sfix(16)  OutScaling=2^0
  Constant2 : xbsIndex_r4/Constant  arith_type=Unsigned  const=(2^CounterBits)-10  n_bits=CounterBits + 1  bin_pt=0  explicit_period=on  period=1  equ=P=C  opselect=C  inp2=PCIN>>17  opr=+  inp1=P  carry=CIN  dbl_ovrd=off  block_type=constant
  Counter3 : xbsIndex_r4/Counter  cnt_type=Free Running  cnt_to=1023  operation=Up  start_count=0  cnt_by_val=1  arith_type=Unsigned  n_bits=CounterBits + 1  bin_pt=0  load_pin=off  rst=on  en=on  explicit_period=on  period=1  dbl_ovrd=off  use_behavioral_HDL=off  implementation=Fabric  use_rpm=on  block_type=counter
      settings: xl_area=[0, 0, 0, 0, 0, 0, 0]  block_version=9.1.01
  Inverter : xbsIndex_r4/Inverter  en=off  latency=0  dbl_ovrd=off  block_type=inv
      settings: xl_area=[0, 0, 0, 0, 0, 0, 0]  block_version=9.1.01
  Inverter1 : xbsIndex_r4/Inverter  en=off  latency=0  dbl_ovrd=off  block_type=inv
      settings: xl_area=[0, 0, 0, 0, 0, 0, 0]  block_version=9.1.01
  Logical1 : xbsIndex_r4/Logical  logical_function=AND  inputs=2  en=off  latency=0  precision=Full  arith_type=Unsigned  n_bits=8  bin_pt=2  align_bp=on  dbl_ovrd=off  block_type=logical
      settings: xl_area=[0, 0, 0, 0, 0, 0, 0]  block_version=9.1.01
  Logical5 : xbsIndex_r4/Logical  logical_function=AND  inputs=2  en=off  latency=0  precision=Full  arith_type=Unsigned  n_bits=8  bin_pt=2  align_bp=on  dbl_ovrd=off  block_type=logical
      settings: xl_area=[0, 0, 0, 0, 0, 0, 0]  block_version=9.1.01
  Relational3 : xbsIndex_r4/Relational  mode=a>=b  en=off  latency=0  dbl_ovrd=off  block_type=relational
      settings: xl_area=[0, 0, 0, 0, 0, 0, 0]  block_version=10.1.3
  enable : xbsIndex_r4/Slice  nbits=CounterBits  boolean_output=off  mode=Lower Bit Location + Width  bit1=0  base1=LSB of Input  bit0=0  base0=LSB of Input  dbl_ovrd=off  block_type=slice
      settings: infoedit="Extracts a given range of bits from each input sample and presents it at the output.  The output type is ordinarily unsigned with binary point at zero, but can be Boolean when the slice is one bit wide.<P><P>Hardware notes: In hardware this block costs nothing."  block_version=9.1.01
  enable1 : xbsIndex_r4/Slice  nbits=1  boolean_output=on  mode=Upper Bit Location + Width  bit1=0  base1=MSB of Input  bit0=0  base0=LSB of Input  dbl_ovrd=off  block_type=slice
      settings: infoedit="Extracts a given range of bits from each input sample and presents it at the output.  The output type is ordinarily unsigned with binary point at zero, but can be Boolean when the slice is one bit wide.<P><P>Hardware notes: In hardware this block costs nothing."  block_version=9.1.01
  addr : Outport  OutDataType=sfix(16)  OutScaling=2^0
  we : Outport  Port=2  OutDataType=sfix(16)  OutScaling=2^0
  afull : Outport  Port=3  OutDataType=sfix(16)  OutScaling=2^0
  wires:
  Inverter1/1 -> Logical5/2
  enable/1 -> addr/1
  rst/1 -> Counter3/1, Inverter/1
  Logical5/1 -> Counter3/2, Logical1/2
  en/1 -> Logical5/1
  enable1/1 -> Inverter1/1
  Counter3/1 -> enable/1, enable1/1, Relational3/1
  Inverter/1 -> Logical1/1
  Logical1/1 -> we/1
  Constant2/1 -> Relational3/2
  Relational3/1 -> afull/1
